simulink model "SModel"  (R2020b)
settings: Solver=FixedStepAuto  StartTime=0.0  StopTime=20  FixedStep=0.01  RelTol=1e-3
values from neighbouring files (symbols this model uses):
  g = 9.81    [LoadParameters.m]    (also in sfun_balrob_long_dyn.m)
  gbox = block.DialogPrm(4).Data    [sfun_balrob_long_dyn.m]
  ms22g = 1/g    (= 0.101936799185)    [LoadParameters.m]
  Nu = X(5)    [LoadParameters.m]
  Nx = X(1:4)    [LoadParameters.m]
  Ts = 1e-2    (= 0.01)    [LoadParameters.m]
  wheel = block.DialogPrm(5).Data    [sfun_balrob_long_dyn.m]
undefined symbols (not defined in the file or in its folder): DiscIntNeverNeededParam, drv, lqr_integral, lqr_nominal, sens, stvar_est
settings Model: Creator=Utente  LastModifiedBy=Utente

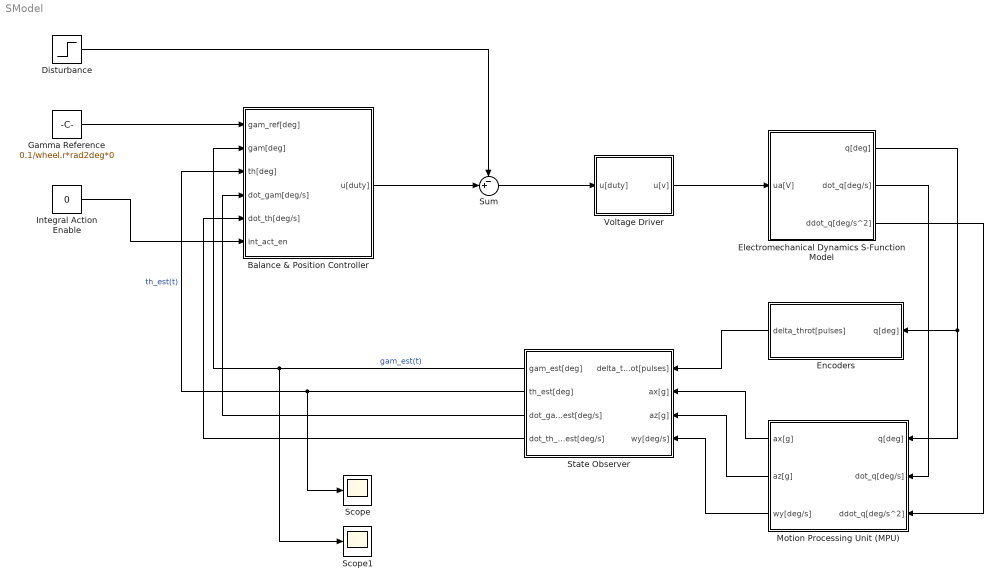
== system SModel ==
  Balance & Position Controller : Subsystem
  Disturbance : Step  Time=20  After=5.0/drv.duty2V  SampleTime=0
  Electromechanical Dynamics S-Function Model : Subsystem
  Encoders : Subsystem
  Gamma Reference : Constant  Value=0.1/wheel.r*rad2deg*0
  Integral Action Enable : Constant  Value=0
  Motion Processing Unit (MPU) : Subsystem
  Scope : Scope
  Scope1 : Scope
  State Observer : Subsystem
  Sum : Sum  Inputs=-+|
  Voltage Driver : Subsystem
  wires:
  Voltage Driver/1(u[v]) -> Electromechanical Dynamics S-Function Model/1(ua[V])
  Electromechanical Dynamics S-Function Model/2(dot_q[deg/s]) -> Motion Processing Unit (MPU)/2(dot_q[deg/s])
  Electromechanical Dynamics S-Function Model/3(ddot_q[deg/s^2]) -> Motion Processing Unit (MPU)/3(ddot_q[deg/s^2])
  Encoders/1(delta_throt[pulses]) -> State Observer/1(delta_throt[pulses])
  Motion Processing Unit (MPU)/3(wy[deg/s]) -> State Observer/4(wy[deg/s])
  Motion Processing Unit (MPU)/2(az[g]) -> State Observer/3(az[g])
  Motion Processing Unit (MPU)/1(ax[g]) -> State Observer/2(ax[g])
  Balance & Position Controller/1(u[duty]) -> Sum/2
  Disturbance/1 -> Sum/1
  State Observer/4(dot_th_est[deg/s]) -> Balance & Position Controller/5(dot_th[deg/s])
  State Observer/3(dot_gam_est[deg/s]) -> Balance & Position Controller/4(dot_gam[deg/s])
  State Observer/2(th_est[deg]) -> Scope/1, Balance & Position Controller/3(th[deg])  "th_est(t)"
  State Observer/1(gam_est[deg]) -> Scope1/1, Balance & Position Controller/2(gam[deg])  "gam_est(t)"
  Gamma Reference/1 -> Balance & Position Controller/1(gam_ref[deg])
  Electromechanical Dynamics S-Function Model/1(q[deg]) -> Motion Processing Unit (MPU)/1(q[deg]), Encoders/1(q[deg])
  Sum/1 -> Voltage Driver/1(u[duty])
  Integral Action Enable/1 -> Balance & Position Controller/6(int_act_en)

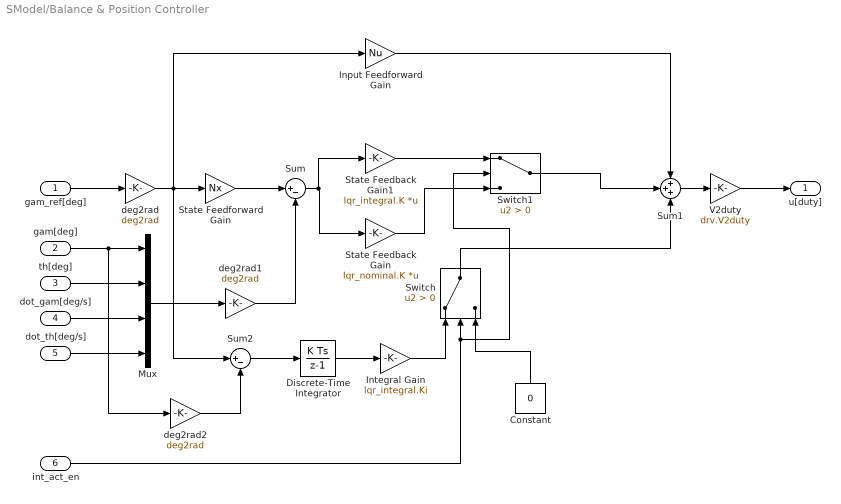
== system SModel/Balance & Position Controller ==
  gam_ref[deg] : Inport
  gam[deg] : Inport  Port=2
  th[deg] : Inport  Port=3
  dot_gam[deg/s] : Inport  Port=4
  dot_th[deg/s] : Inport  Port=5
  int_act_en : Inport  Port=6
  Constant : Constant  Value=0
  Discrete-Time Integrator : DiscreteIntegrator  SampleTime=Ts  ICPrevOutput=DiscIntNeverNeededParam  ICPrevScaledInput=DiscIntNeverNeededParam
  Input Feedforward Gain : Gain  Gain=Nu
  Integral Gain : Gain  Gain=lqr_integral.Ki
  Mux : Mux
  State Feedback Gain : Gain  Gain=lqr_nominal.K  Multiplication=Matrix(K*u)
  State Feedback Gain1 : Gain  Gain=lqr_integral.K  Multiplication=Matrix(K*u)
  State Feedforward Gain : Gain  Gain=Nx
  Sum : Sum  Inputs=|+-
  Sum1 : Sum  Inputs=+++
  Sum2 : Sum  Inputs=|+-
  Switch : Switch  Criteria=u2 > Threshold
  Switch1 : Switch  Criteria=u2 > Threshold
  V2duty : Gain  Gain=drv.V2duty
  deg2rad : Gain  Gain=deg2rad
  deg2rad1 : Gain  Gain=deg2rad
  deg2rad2 : Gain  Gain=deg2rad
  u[duty] : Outport
  wires:
  Mux/1 -> deg2rad1/1
  Sum1/1 -> V2duty/1
  th[deg]/1 -> Mux/2
  deg2rad/1 -> Sum2/1, Input Feedforward Gain/1, State Feedforward Gain/1
  dot_gam[deg/s]/1 -> Mux/3
  Input Feedforward Gain/1 -> Sum1/1
  V2duty/1 -> u[duty]/1
  gam_ref[deg]/1 -> deg2rad/1
  gam[deg]/1 -> deg2rad2/1, Mux/1
  dot_th[deg/s]/1 -> Mux/4
  State Feedforward Gain/1 -> Sum/1
  deg2rad1/1 -> Sum/2
  Sum/1 -> State Feedback Gain1/1, State Feedback Gain/1
  Sum2/1 -> Discrete-Time Integrator/1
  deg2rad2/1 -> Sum2/2
  Discrete-Time Integrator/1 -> Integral Gain/1
  Integral Gain/1 -> Switch/1
  Constant/1 -> Switch/3
  int_act_en/1 -> Switch1/2, Switch/2
  State Feedback Gain/1 -> Switch1/3
  Switch1/1 -> Sum1/2
  State Feedback Gain1/1 -> Switch1/1
  Switch/1 -> Sum1/3

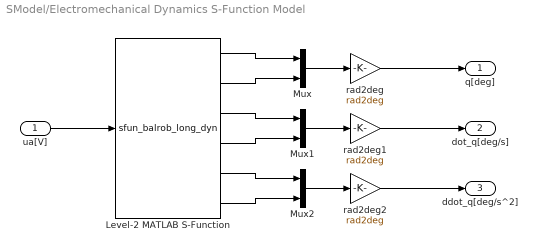
== system SModel/Electromechanical Dynamics S-Function Model ==
  ua[V] : Inport
  Level-2 MATLAB S-Function : M-S-Function  FunctionName=sfun_balrob_long_dyn  Parameters=x02, body, mot, gbox, wheel
  Mux : Mux  Inputs=2
  Mux1 : Mux  Inputs=2
  Mux2 : Mux  Inputs=2
  rad2deg : Gain  Gain=rad2deg
  rad2deg1 : Gain  Gain=rad2deg
  rad2deg2 : Gain  Gain=rad2deg
  q[deg] : Outport
  dot_q[deg/s] : Outport  Port=2
  ddot_q[deg/s^2] : Outport  Port=3
  wires:
  Level-2 MATLAB S-Function/6 -> Mux2/2
  Level-2 MATLAB S-Function/4 -> Mux1/2
  rad2deg1/1 -> dot_q[deg/s]/1
  ua[V]/1 -> Level-2 MATLAB S-Function/1
  Mux1/1 -> rad2deg1/1
  rad2deg/1 -> q[deg]/1
  Level-2 MATLAB S-Function/2 -> Mux/2
  Level-2 MATLAB S-Function/5 -> Mux2/1
  rad2deg2/1 -> ddot_q[deg/s^2]/1
  Level-2 MATLAB S-Function/3 -> Mux1/1
  Mux/1 -> rad2deg/1
  Mux2/1 -> rad2deg2/1
  Level-2 MATLAB S-Function/1 -> Mux/1

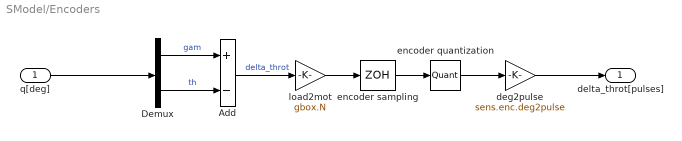
== system SModel/Encoders ==
  q[deg] : Inport
  Add : Sum  Inputs=+-
  Demux : Demux  Outputs=2
  deg2pulse : Gain  Gain=sens.enc.deg2pulse
  encoder quantization : Quantizer  QuantizationInterval=sens.enc.pulse2deg
  encoder sampling : ZeroOrderHold  SampleTime=Ts
  load2mot : Gain  Gain=gbox.N
  delta_throt[pulses] : Outport
  wires:
  Add/1 -> load2mot/1  "delta_throt"
  encoder sampling/1 -> encoder quantization/1
  load2mot/1 -> encoder sampling/1
  encoder quantization/1 -> deg2pulse/1
  Demux/2 -> Add/2  "th"
  deg2pulse/1 -> delta_throt[pulses]/1
  q[deg]/1 -> Demux/1
  Demux/1 -> Add/1  "gam"

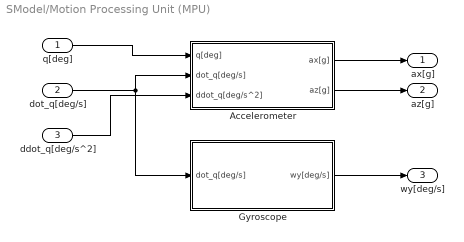
== system SModel/Motion Processing Unit (MPU) ==
  q[deg] : Inport
  dot_q[deg/s] : Inport  Port=2
  ddot_q[deg/s^2] : Inport  Port=3
  Accelerometer : Subsystem
  Gyroscope : Subsystem
  ax[g] : Outport
  az[g] : Outport  Port=2
  wy[deg/s] : Outport  Port=3
  wires:
  ddot_q[deg/s^2]/1 -> Accelerometer/3(ddot_q[deg/s^2])
  Accelerometer/1(ax[g]) -> ax[g]/1
  q[deg]/1 -> Accelerometer/1("q[deg] ")
  dot_q[deg/s]/1 -> Gyroscope/1("dot_q[deg/s] "), Accelerometer/2(dot_q[deg/s])
  Gyroscope/1(wy[deg/s]) -> wy[deg/s]/1
  Accelerometer/2(az[g]) -> az[g]/1

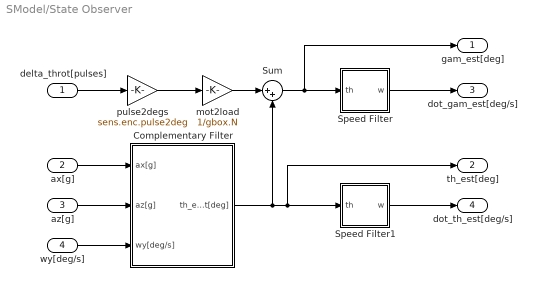
== system SModel/State Observer ==
  delta_throt[pulses] : Inport
  ax[g] : Inport  Port=2
  az[g] : Inport  Port=3
  wy[deg/s] : Inport  Port=4
  Complementary Filter : Subsystem
  Speed Filter : Subsystem
  Speed Filter1 : Subsystem
  Sum : Sum  Inputs=|++
  mot2load : Gain  Gain=1/gbox.N
  pulse2degs : Gain  Gain=sens.enc.pulse2deg
  gam_est[deg] : Outport
  th_est[deg] : Outport  Port=2
  dot_gam_est[deg/s] : Outport  Port=3
  dot_th_est[deg/s] : Outport  Port=4
  wires:
  Complementary Filter/1(th_est[deg]) -> th_est[deg]/1, Speed Filter1/1(th), Sum/2
  delta_throt[pulses]/1 -> pulse2degs/1
  ax[g]/1 -> Complementary Filter/1(ax[g])
  az[g]/1 -> Complementary Filter/2(az[g])
  mot2load/1 -> Sum/1
  wy[deg/s]/1 -> Complementary Filter/3(wy[deg/s])
  Speed Filter/1(w) -> dot_gam_est[deg/s]/1
  Speed Filter1/1(w) -> dot_th_est[deg/s]/1
  pulse2degs/1 -> mot2load/1
  Sum/1 -> gam_est[deg]/1, Speed Filter/1(th)

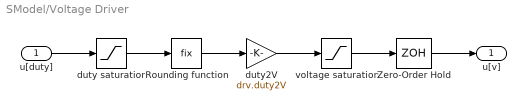
== system SModel/Voltage Driver ==
  u[duty] : Inport
  Rounding function : Rounding  Operator=fix
  Zero-Order Hold : ZeroOrderHold  SampleTime=Ts
  duty saturation : Saturate  UpperLimit=drv.dutymax  LowerLimit=-drv.dutymax
  duty2V : Gain  Gain=drv.duty2V
  voltage saturation : Saturate  UpperLimit=drv.Vbus  LowerLimit=-drv.Vbus
  u[v] : Outport
  wires:
  Zero-Order Hold/1 -> u[v]/1
  u[duty]/1 -> duty saturation/1
  duty saturation/1 -> Rounding function/1
  voltage saturation/1 -> Zero-Order Hold/1
  duty2V/1 -> voltage saturation/1
  Rounding function/1 -> duty2V/1

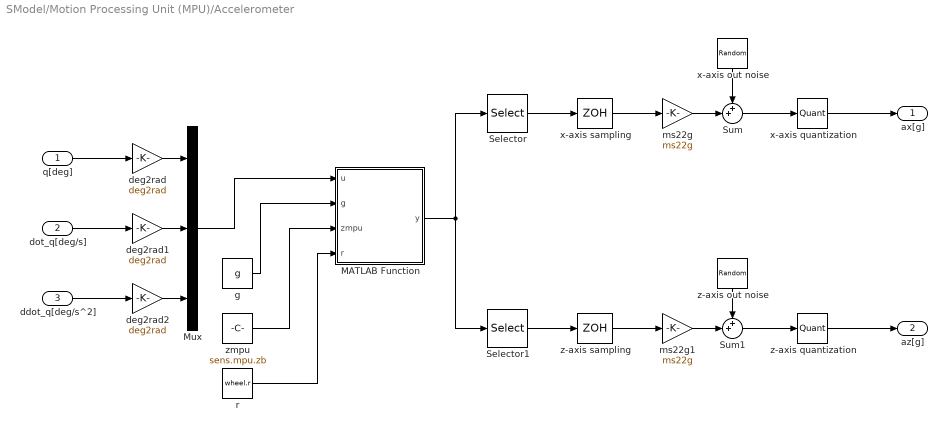
== system SModel/Motion Processing Unit (MPU)/Accelerometer ==
  "q[deg] " : Inport
  dot_q[deg/s] : Inport  Port=2
  ddot_q[deg/s^2] : Inport  Port=3
  MATLAB Function : MATLAB Function  TreatAsAtomicUnit=on
  Mux : Mux  Inputs=3
  Selector : Selector  InputPortWidth=2  IndexOptions=Index vector (dialog)  Indices=1  OutputSizes=1
  Selector1 : Selector  InputPortWidth=2  IndexOptions=Index vector (dialog)  Indices=2  OutputSizes=1
  Sum : Sum  Inputs=++|
  Sum1 : Sum  Inputs=++|
  deg2rad : Gain  Gain=deg2rad
  deg2rad1 : Gain  Gain=deg2rad
  deg2rad2 : Gain  Gain=deg2rad
  g : Constant  Value=g
  ms22g : Gain  Gain=ms22g
  ms22g1 : Gain  Gain=ms22g
  r : Constant  Value=wheel.r
  x-axis out noise : RandomNumber  Variance=sens.mpu.acc.noisevar  SampleTime=0.1
  x-axis quantization : Quantizer  QuantizationInterval=sens.mpu.acc.LSB2g
  x-axis sampling : ZeroOrderHold  SampleTime=-1
  z-axis out noise : RandomNumber  Variance=sens.mpu.acc.noisevar  SampleTime=0.1
  z-axis quantization : Quantizer  QuantizationInterval=sens.mpu.acc.LSB2g
  z-axis sampling : ZeroOrderHold  SampleTime=-1
  zmpu : Constant  Value=sens.mpu.zb
  ax[g] : Outport
  az[g] : Outport  Port=2
  wires:
  x-axis sampling/1 -> ms22g/1
  z-axis quantization/1 -> az[g]/1
  deg2rad1/1 -> Mux/2
  x-axis quantization/1 -> ax[g]/1
  ms22g/1 -> Sum/2
  dot_q[deg/s]/1 -> deg2rad1/1
  ms22g1/1 -> Sum1/2
  Sum/1 -> x-axis quantization/1
  Sum1/1 -> z-axis quantization/1
  z-axis out noise/1 -> Sum1/1
  z-axis sampling/1 -> ms22g1/1
  x-axis out noise/1 -> Sum/1
  Mux/1 -> MATLAB Function/1(u)
  Selector1/1 -> z-axis sampling/1
  deg2rad2/1 -> Mux/3
  ddot_q[deg/s^2]/1 -> deg2rad2/1
  deg2rad/1 -> Mux/1
  "q[deg] "/1 -> deg2rad/1
  g/1 -> MATLAB Function/2(g)
  zmpu/1 -> MATLAB Function/3(zmpu)
  r/1 -> MATLAB Function/4(r)
  Selector/1 -> x-axis sampling/1
  MATLAB Function/1(y) -> Selector1/1, Selector/1

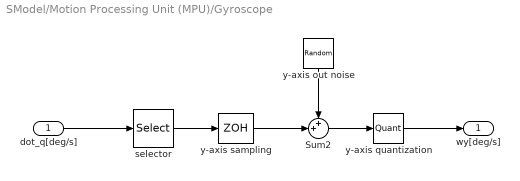
== system SModel/Motion Processing Unit (MPU)/Gyroscope ==
  "dot_q[deg/s] " : Inport
  Sum2 : Sum  Inputs=++|
  selector : Selector  InputPortWidth=2  IndexOptions=Index vector (dialog)  Indices=[2]  OutputSizes=1
  y-axis out noise : RandomNumber  Variance=sens.mpu.gyro.noisevar  SampleTime=0.1
  y-axis quantization : Quantizer  QuantizationInterval=sens.mpu.gyro.LSB2degs
  y-axis sampling : ZeroOrderHold  SampleTime=-1
  wy[deg/s] : Outport
  wires:
  Sum2/1 -> y-axis quantization/1
  y-axis out noise/1 -> Sum2/1
  y-axis quantization/1 -> wy[deg/s]/1
  selector/1 -> y-axis sampling/1
  y-axis sampling/1 -> Sum2/2
  "dot_q[deg/s] "/1 -> selector/1

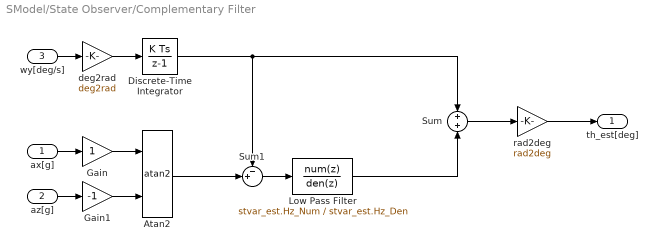
== system SModel/State Observer/Complementary Filter ==
  ax[g] : Inport
  az[g] : Inport  Port=2
  wy[deg/s] : Inport  Port=3
  Atan2 : Trigonometry  Operator=atan2
  Discrete-Time Integrator : DiscreteIntegrator  SampleTime=Ts  ICPrevOutput=DiscIntNeverNeededParam  ICPrevScaledInput=DiscIntNeverNeededParam
  Gain : Gain
  Gain1 : Gain  Gain=-1
  "Low Pass Filter " : DiscreteTransferFcn  Numerator=stvar_est.Hz_Num  Denominator=stvar_est.Hz_Den
  Sum : Sum  Inputs=+|+
  Sum1 : Sum  Inputs=-+|
  deg2rad : Gain  Gain=deg2rad
  rad2deg : Gain  Gain=rad2deg
  th_est[deg] : Outport
  wires:
  ax[g]/1 -> Gain/1
  deg2rad/1 -> Discrete-Time Integrator/1
  wy[deg/s]/1 -> deg2rad/1
  Atan2/1 -> Sum1/2
  Gain1/1 -> Atan2/2
  Gain/1 -> Atan2/1
  az[g]/1 -> Gain1/1
  rad2deg/1 -> th_est[deg]/1
  Sum/1 -> rad2deg/1
  Discrete-Time Integrator/1 -> Sum1/1, Sum/1
  Sum1/1 -> "Low Pass Filter "/1
  "Low Pass Filter "/1 -> Sum/2

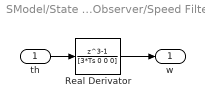
== system SModel/State Observer/Speed Filter ==
  th : Inport
  Real Derivator : DiscreteTransferFcn  Numerator=[1 0 0 -1]  Denominator=[3*Ts 0 0 0]  SampleTime=Ts
  w : Outport
  wires:
  Real Derivator/1 -> w/1
  th/1 -> Real Derivator/1

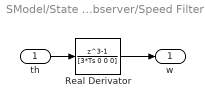
== system SModel/State Observer/Speed Filter1 ==
  th : Inport
  Real Derivator : DiscreteTransferFcn  Numerator=[1 0 0 -1]  Denominator=[3*Ts 0 0 0]  SampleTime=Ts
  w : Outport
  wires:
  Real Derivator/1 -> w/1
  th/1 -> Real Derivator/1

== matlab function SModel/Motion Processing Unit (MPU)/Accelerometer/MATLAB Function ==
  data: u input; y output; g input; zmpu input; r input
function y = fcn(u, g, zmpu, r)
theta = u(2);
dot_theta = u(4);
ddot_theta = u(6);
ddot_gamma = u(5);
y = [r*ddot_gamma*cos(theta)+zmpu*ddot_theta+g*sin(theta);r*ddot_gamma*sin(theta)-zmpu*dot_theta*dot_theta-g*cos(theta)];
